simulink model "path_select_sl"  (R2019a)
settings: Solver=VariableStepAuto  StartTime=0.0  StopTime=inf  RelTol=1e-3
model workspace (MAT data in the model file):
  SL_ROS_VariableLengthArrays_MaxSizes.CommonInfo.ArrayTruncateAction = 'EmitWarning'
  SL_ROS_VariableLengthArrays_MaxSizes.MsgTypeMap = containers.Map
  SL_ROS_VariableLengthArrays_MaxSizes.MsgTypeMap.serialization.keys = {'autoware_msgs/Lane', 'autoware_msgs/LaneArray', 'autoware_msgs/lane'}
  SL_ROS_VariableLengthArrays_MaxSizes.MsgTypeMap.serialization.values{1}.PropertyName = 'Waypoints'
  SL_ROS_VariableLengthArrays_MaxSizes.MsgTypeMap.serialization.values{1}.DataType = 'autoware_msgs/Waypoint'
  SL_ROS_VariableLengthArrays_MaxSizes.MsgTypeMap.serialization.values{1}.MaxLength = 2587
  SL_ROS_VariableLengthArrays_MaxSizes.MsgTypeMap.serialization.values{2}.PropertyName = 'Lanes'
  SL_ROS_VariableLengthArrays_MaxSizes.MsgTypeMap.serialization.values{2}.DataType = 'autoware_msgs/Lane'
  SL_ROS_VariableLengthArrays_MaxSizes.MsgTypeMap.serialization.values{2}.MaxLength = 1
  SL_ROS_VariableLengthArrays_MaxSizes.MsgTypeMap.serialization.values{3}.PropertyName = 'Waypoints'
  SL_ROS_VariableLengthArrays_MaxSizes.MsgTypeMap.serialization.values{3}.DataType = 'autoware_msgs/waypoint'
  SL_ROS_VariableLengthArrays_MaxSizes.MsgTypeMap.serialization.values{3}.MaxLength = 101
  SL_ROS_VariableLengthArrays_MaxSizes.MsgTypeMap.serialization.uniformity = 0
  SL_ROS_VariableLengthArrays_MaxSizes.MsgTypeMap.serialization.keyType = 'char'
  SL_ROS_VariableLengthArrays_MaxSizes.MsgTypeMap.serialization.valueType = 'any'
libraries: robotlib x2
settings Model: Creator=handai  LastModifiedBy=root
settings DataIOCC: ReturnWorkspaceOutputs=off
settings DebuggingCC: ArithmeticOperatorsInVariantConditions=warning

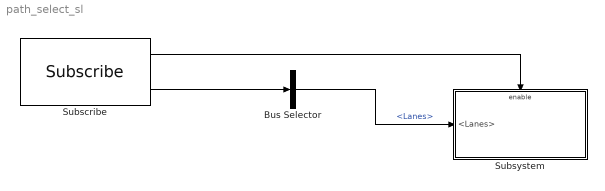
== system path_select_sl ==
  Bus Selector : BusSelector  OutputSignals=Lanes
  Subscribe : robotlib/Subscribe  topicSource=Specify your own  topic=/traffic_waypoints_array  messageType=autoware_msgs/LaneArray  sampleTime=-1  messageQueueLength=1
      settings: SourceProductBaseCode=RO
  Subsystem : Subsystem
  wires:
  Subscribe/1 -> Subsystem/Enable
  Subscribe/2 -> Bus Selector/1
  Bus Selector/1 -> Subsystem/1(<Lanes>)  "<Lanes>"

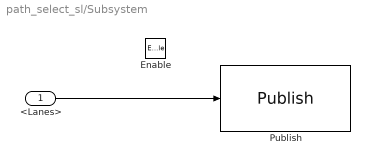
== system path_select_sl/Subsystem ==
  <Lanes> : Inport
  Enable : EnablePort
  Publish : robotlib/Publish  topicSource=Specify your own  topic=/base_waypoints  messageType=autoware_msgs/Lane  messageQueueLength=1
      settings: SourceProductBaseCode=RO
  wires:
  <Lanes>/1 -> Publish/1
